simulink model "g729_enc_test_bench"  (R2013b)
settings: Solver=ode45  StartTime=0.0  StopTime=10000  RelTol=1e-3
PreLoadFcn:
  | g729_init
values from neighbouring files (symbols this model uses):
  fpga_up_rate = 20    [g729_init.m]
libraries: xbsIndex_r4 x50
settings Model: Creator=asubbiah  LastModifiedBy=asubbiah

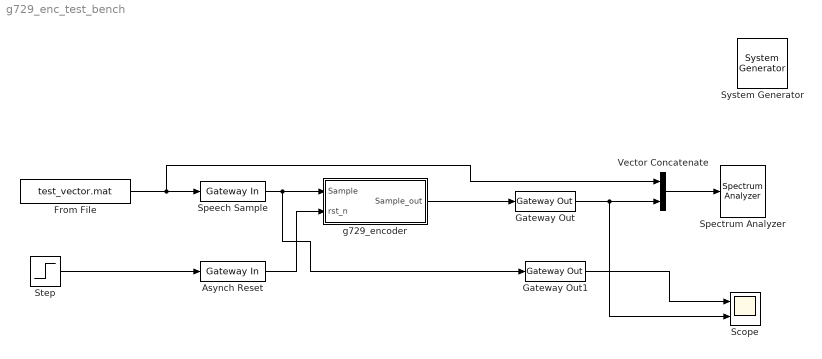
== system g729_enc_test_bench ==
  " System Generator" : xbsIndex_r4/ System Generator  Tag=genX  xilinxfamily=kintex7  part=xc7k325t  speed=-3  package=fbg676  synthesis_tool=Vivado  clock_wrapper=Clock Enables  directory=./netlist  proj_type=Vivado  Synth_file=Vivado Synthesis Defaults  Impl_file=Vivado Implementation Defaults  testbench=off  simulink_period=1/fpga_up_rate*2  sysclk_period=100  dcm_input_clock_period=10  incr_netlist=off  trim_vbits=Everywhere in SubSystem  dbl_ovrd=According to Block Masks  core_generation=According to Block Masks  run_coregen=off  deprecated_control=off  eval_field=0  block_type=sysgen
  Asynch Reset : xbsIndex_r4/Gateway In  gui_display_data_type=Boolean  arith_type=Boolean  n_bits=fixed_point  bin_pt=fixed_point_frac  preci_type=Single  exp_width=8  frac_width=24  quantization="Round  (unbiased: +/- Inf)"  overflow=Saturate  period=1  UseAsADC=off  ADCChannel='1'  interface=None  automatic_assignment=on  address_offset=hex2dec('00')  intf_description=''  timing_constraint=None  locs_specified=off  LOCs={}  io_standard={}  inherit_from_input=off  hdl_port=on  dbl_ovrd=off  block_type=gatewayin
  From File : FromFile  FileName=test_vector.mat  SampleTime=64
  Gateway Out : xbsIndex_r4/Gateway Out  inherit_from_input=off  hdl_port=on  rows=1  columns=1  UseAsDAC=off  DACChannel='1'  interface=None  automatic_assignment=on  address_offset=hex2dec('00')  intf_description=''  timing_constraint=None  locs_specified=off  LOCs={}  io_standard={}  block_type=gatewayout
  Gateway Out1 : xbsIndex_r4/Gateway Out  inherit_from_input=off  hdl_port=on  rows=1  columns=1  UseAsDAC=off  DACChannel='1'  interface=None  automatic_assignment=on  address_offset=hex2dec('00')  intf_description=''  timing_constraint=None  locs_specified=off  LOCs={}  io_standard={}  block_type=gatewayout
  Scope : Scope  NumInputPorts=2
      settings: YMin=-0.75~-1.2  YMax=0.75~0.2  MaxDataPoints=50000
  Spectrum Analyzer : SpectrumAnalyzer
      settings: CopyFcn=scopeextensions.ScopeBlock.onCoreBlockCopy(gcbh);  DeleteFcn=scopeextensions.ScopeBlock.callback(gcbh, 'onBlockDelete');  PreSaveFcn=scopeextensions.ScopeBlock.callback(gcbh, 'onModelSave');  NameChangeFcn=scopeextensions.ScopeBlock.callback(gcbh, 'onBlockRename');  DestroyFcn=scopeextensions.ScopeBlock.onBlockDestroy(gcbh)  CloseFcn=scopeextensions.ScopeBlock.callback(gcbh, 'onBlockClose');  PreDeleteFcn=scopeextensions.ScopeBlock.callback(gcbh, 'onBlockPreDelete');
  Speech Sample : xbsIndex_r4/Gateway In  gui_display_data_type=Fixed-point  arith_type="Signed  (2's comp)"  n_bits=fixed_point  bin_pt=fixed_point_frac  preci_type=Single  exp_width=8  frac_width=24  quantization="Round  (unbiased: +/- Inf)"  overflow=Saturate  period=1  UseAsADC=off  ADCChannel='1'  interface=None  automatic_assignment=on  address_offset=hex2dec('00')  intf_description=''  timing_constraint=None  locs_specified=off  LOCs={}  io_standard={}  inherit_from_input=off  hdl_port=on  dbl_ovrd=off  block_type=gatewayin
  Step : Step  SampleTime=0
  Vector Concatenate : Concatenate  Mode=Multidimensional array  ConcatenateDimension=2
  g729_encoder : Subsystem
  wires:
  Step/1 -> Asynch Reset/1
  From File/1 -> Vector Concatenate/1, Speech Sample/1
  Speech Sample/1 -> Gateway Out1/1, g729_encoder/1(Sample)
  Asynch Reset/1 -> g729_encoder/2(rst_n)
  g729_encoder/1(Sample_out) -> Gateway Out/1
  Gateway Out/1 -> Scope/2, Vector Concatenate/2
  Vector Concatenate/1 -> Spectrum Analyzer/1
  Gateway Out1/1 -> Scope/1

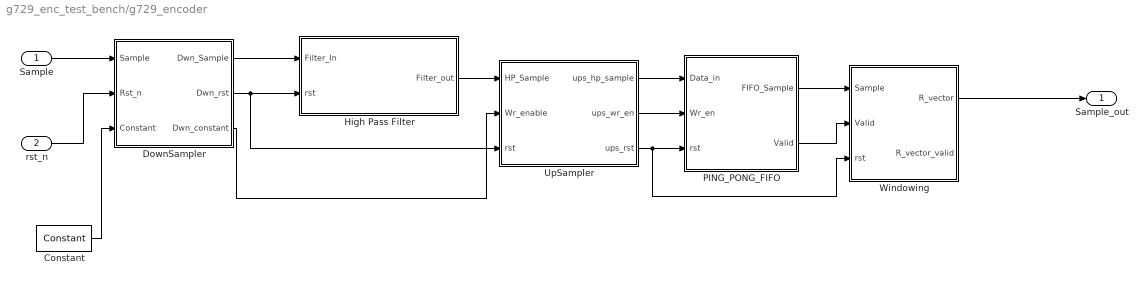
== system g729_enc_test_bench/g729_encoder ==
  Sample : Inport
  rst_n : Inport  Port=2
  Constant : xbsIndex_r4/Constant  const=1  gui_display_data_type=Boolean  arith_type=Boolean  n_bits=16  bin_pt=14  preci_type=Single  exp_width=8  frac_width=24  explicit_period=on  period=1  equ=P=C  opselect=C  inp2=PCIN>>17  opr=+  inp1=P  carry=CIN  dbl_ovrd=off  block_type=constant
  DownSampler : Subsystem
  High Pass Filter : Subsystem
  PING_PONG_FIFO : Subsystem
  UpSampler : Subsystem
  Windowing : Subsystem
  Sample_out : Outport
  wires:
  Sample/1 -> DownSampler/1(Sample)
  DownSampler/1(Dwn_Sample) -> High Pass Filter/1(Filter_In)
  DownSampler/2(Dwn_rst) -> High Pass Filter/2(rst), UpSampler/3(rst)
  rst_n/1 -> DownSampler/2(Rst_n)
  Constant/1 -> DownSampler/3(Constant)
  High Pass Filter/1(Filter_out) -> UpSampler/1(HP_Sample)
  UpSampler/1(ups_hp_sample) -> PING_PONG_FIFO/1(Data_in)
  UpSampler/2(ups_wr_en) -> PING_PONG_FIFO/2(Wr_en)
  DownSampler/3(Dwn_constant) -> UpSampler/2(Wr_enable)
  UpSampler/3(ups_rst) -> PING_PONG_FIFO/3(rst), Windowing/3(rst)
  PING_PONG_FIFO/1(FIFO_Sample) -> Windowing/1(Sample)
  PING_PONG_FIFO/2(Valid) -> Windowing/2(Valid)
  Windowing/1(R_vector) -> Sample_out/1

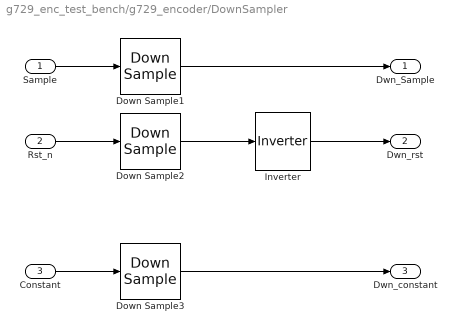
== system g729_enc_test_bench/g729_encoder/DownSampler ==
  Sample : Inport
  Rst_n : Inport  Port=2
  Constant : Inport  Port=3
  Down Sample1 : xbsIndex_r4/Down Sample  sample_ratio=2  sample_phase="Last Value of Frame  (most efficient)"  en=off  rst=off  latency=2  dbl_ovrd=off  block_type=dsamp
  Down Sample2 : xbsIndex_r4/Down Sample  sample_ratio=2  sample_phase="Last Value of Frame  (most efficient)"  en=off  rst=off  latency=2  dbl_ovrd=off  block_type=dsamp
  Down Sample3 : xbsIndex_r4/Down Sample  sample_ratio=2  sample_phase="Last Value of Frame  (most efficient)"  en=off  rst=off  latency=2  dbl_ovrd=off  block_type=dsamp
  Inverter : xbsIndex_r4/Inverter  en=off  latency=0  dbl_ovrd=off  block_type=inv
  Dwn_Sample : Outport
  Dwn_rst : Outport  Port=2
  Dwn_constant : Outport  Port=3
  wires:
  Sample/1 -> Down Sample1/1
  Down Sample1/1 -> Dwn_Sample/1
  Rst_n/1 -> Down Sample2/1
  Down Sample2/1 -> Inverter/1
  Inverter/1 -> Dwn_rst/1
  Constant/1 -> Down Sample3/1
  Down Sample3/1 -> Dwn_constant/1

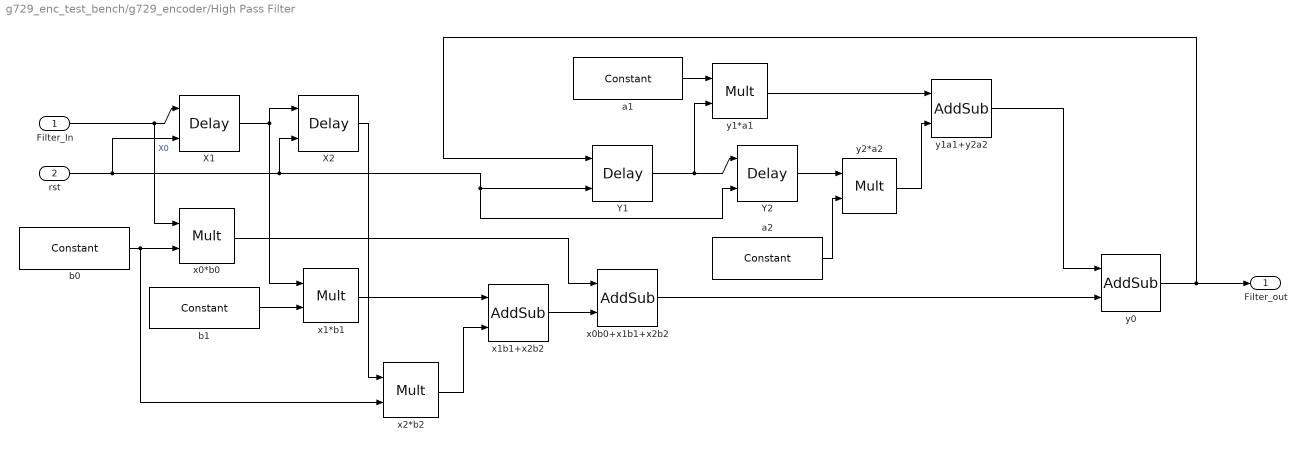
== system g729_enc_test_bench/g729_encoder/High Pass Filter ==
  Filter_In : Inport
  rst : Inport  Port=2
  X1 : xbsIndex_r4/Delay  rst=on  infoeditControl=Selection of Reset will increase slice count due to use of real FFs and instead of SRLs  en=off  latency=1  reg_retiming=off  dbl_ovrd=off  block_type=delay
  X2 : xbsIndex_r4/Delay  rst=on  infoeditControl=Selection of Reset will increase slice count due to use of real FFs and instead of SRLs  en=off  latency=1  reg_retiming=off  dbl_ovrd=off  block_type=delay
  Y1 : xbsIndex_r4/Delay  rst=on  infoeditControl=Selection of Reset will increase slice count due to use of real FFs and instead of SRLs  en=off  latency=1  reg_retiming=off  dbl_ovrd=off  block_type=delay
  Y2 : xbsIndex_r4/Delay  rst=on  infoeditControl=Selection of Reset will increase slice count due to use of real FFs and instead of SRLs  en=off  latency=1  reg_retiming=off  dbl_ovrd=off  block_type=delay
  a1 : xbsIndex_r4/Constant  const=1.9059465  gui_display_data_type=Fixed-point  arith_type=Signed (2's comp)  n_bits=fixed_point  bin_pt=fixed_point_frac  preci_type=Single  exp_width=8  frac_width=24  explicit_period=off  period=1  equ=P=C  opselect=C  inp2=PCIN>>17  opr=+  inp1=P  carry=CIN  dbl_ovrd=off  block_type=constant
  a2 : xbsIndex_r4/Constant  const=-0.91140240  gui_display_data_type=Fixed-point  arith_type=Signed (2's comp)  n_bits=fixed_point  bin_pt=fixed_point_frac  preci_type=Single  exp_width=8  frac_width=24  explicit_period=off  period=1  equ=P=C  opselect=C  inp2=PCIN>>17  opr=+  inp1=P  carry=CIN  dbl_ovrd=off  block_type=constant
  b0 : xbsIndex_r4/Constant  const=0.46363718  gui_display_data_type=Fixed-point  arith_type=Signed (2's comp)  n_bits=fixed_point  bin_pt=fixed_point_frac  preci_type=Single  exp_width=8  frac_width=24  explicit_period=off  period=1  equ=P=C  opselect=C  inp2=PCIN>>17  opr=+  inp1=P  carry=CIN  dbl_ovrd=off  block_type=constant
  b1 : xbsIndex_r4/Constant  const=-0.92724705  gui_display_data_type=Fixed-point  arith_type=Signed (2's comp)  n_bits=fixed_point  bin_pt=fixed_point_frac  preci_type=Single  exp_width=8  frac_width=24  explicit_period=off  period=1  equ=P=C  opselect=C  inp2=PCIN>>17  opr=+  inp1=P  carry=CIN  dbl_ovrd=off  block_type=constant
  x0*b0 : xbsIndex_r4/Mult  precision=User Defined  arith_type="Signed  (2's comp)"  n_bits=fixed_point  bin_pt=fixed_point_frac  quantization=Truncate  overflow=Wrap  en=off  latency=0  use_behavioral_HDL=off  opt=Speed  use_embedded=on  optimum_pipeline=off  pipeline=on  dbl_ovrd=off  use_rpm=on  placement_style=Triangular  block_type=mult
  x0b0+x1b1+x2b2 : xbsIndex_r4/AddSub  mode=Addition  use_carryin=off  use_carryout=off  en=off  latency=0  precision=Full  arith_type=Unsigned  n_bits=16  bin_pt=14  quantization=Truncate  overflow=Wrap  use_behavioral_HDL=off  hw_selection=Fabric  pipelined=on  dbl_ovrd=off  block_type=addsub
  x1*b1 : xbsIndex_r4/Mult  precision=User Defined  arith_type="Signed  (2's comp)"  n_bits=fixed_point  bin_pt=fixed_point_frac  quantization=Truncate  overflow=Wrap  en=off  latency=0  use_behavioral_HDL=off  opt=Speed  use_embedded=on  optimum_pipeline=off  pipeline=on  dbl_ovrd=off  use_rpm=on  placement_style=Triangular  block_type=mult
  x1b1+x2b2 : xbsIndex_r4/AddSub  mode=Addition  use_carryin=off  use_carryout=off  en=off  latency=0  precision=Full  arith_type=Unsigned  n_bits=16  bin_pt=14  quantization=Truncate  overflow=Wrap  use_behavioral_HDL=off  hw_selection=Fabric  pipelined=on  dbl_ovrd=off  block_type=addsub
  x2*b2 : xbsIndex_r4/Mult  precision=User Defined  arith_type="Signed  (2's comp)"  n_bits=fixed_point  bin_pt=fixed_point_frac  quantization=Truncate  overflow=Wrap  en=off  latency=0  use_behavioral_HDL=off  opt=Speed  use_embedded=on  optimum_pipeline=off  pipeline=on  dbl_ovrd=off  use_rpm=on  placement_style=Triangular  block_type=mult
  y0 : xbsIndex_r4/AddSub  mode=Addition  use_carryin=off  use_carryout=off  en=off  latency=0  precision=Full  arith_type=Unsigned  n_bits=16  bin_pt=14  quantization=Truncate  overflow=Wrap  use_behavioral_HDL=off  hw_selection=Fabric  pipelined=on  dbl_ovrd=off  block_type=addsub
  y1*a1 : xbsIndex_r4/Mult  precision=User Defined  arith_type="Signed  (2's comp)"  n_bits=fixed_point  bin_pt=fixed_point_frac  quantization=Truncate  overflow=Wrap  en=off  latency=0  use_behavioral_HDL=off  opt=Speed  use_embedded=on  optimum_pipeline=off  pipeline=on  dbl_ovrd=off  use_rpm=on  placement_style=Triangular  block_type=mult
  y1a1+y2a2 : xbsIndex_r4/AddSub  mode=Addition  use_carryin=off  use_carryout=off  en=off  latency=0  precision=Full  arith_type=Unsigned  n_bits=16  bin_pt=14  quantization=Truncate  overflow=Wrap  use_behavioral_HDL=off  hw_selection=Fabric  pipelined=on  dbl_ovrd=off  block_type=addsub
  y2*a2 : xbsIndex_r4/Mult  precision=User Defined  arith_type="Signed  (2's comp)"  n_bits=fixed_point  bin_pt=fixed_point_frac  quantization=Truncate  overflow=Wrap  en=off  latency=0  use_behavioral_HDL=off  opt=Speed  use_embedded=on  optimum_pipeline=off  pipeline=on  dbl_ovrd=off  use_rpm=on  placement_style=Triangular  block_type=mult
  Filter_out : Outport
  wires:
  rst/1 -> X1/2, X2/2, Y2/2, Y1/2
  y0/1 -> Filter_out/1, Y1/1
  y1a1+y2a2/1 -> y0/1
  x0b0+x1b1+x2b2/1 -> y0/2
  Y2/1 -> y2*a2/1
  a2/1 -> y2*a2/2
  y2*a2/1 -> y1a1+y2a2/2
  y1*a1/1 -> y1a1+y2a2/1
  a1/1 -> y1*a1/1
  Y1/1 -> y1*a1/2, Y2/1
  x2*b2/1 -> x1b1+x2b2/2
  x1*b1/1 -> x1b1+x2b2/1
  x0*b0/1 -> x0b0+x1b1+x2b2/1
  x1b1+x2b2/1 -> x0b0+x1b1+x2b2/2
  b0/1 -> x0*b0/2, x2*b2/2
  X2/1 -> x2*b2/1
  b1/1 -> x1*b1/2
  X1/1 -> x1*b1/1, X2/1
  Filter_In/1 -> X1/1, x0*b0/1  "X0"

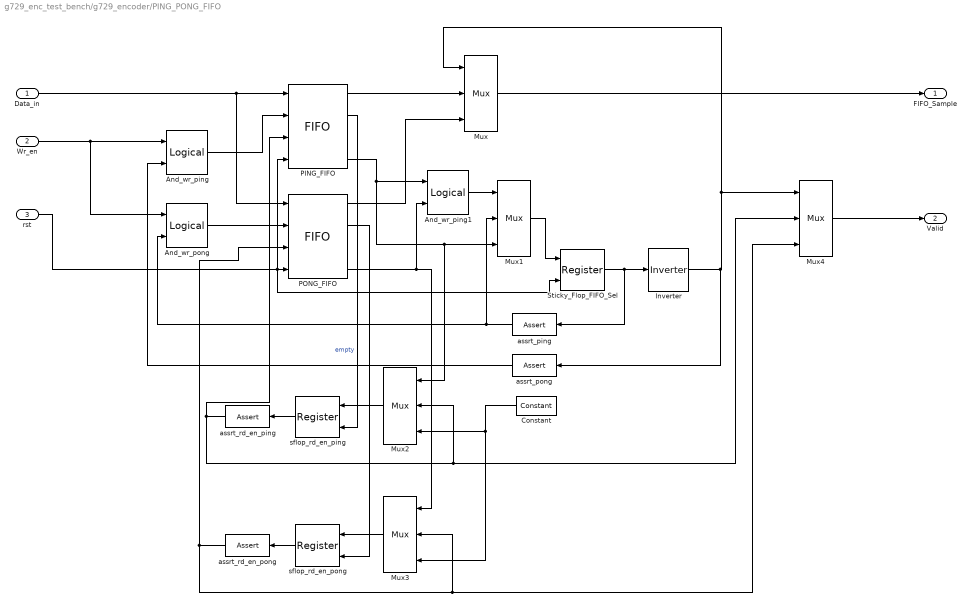
== system g729_enc_test_bench/g729_encoder/PING_PONG_FIFO ==
  Data_in : Inport
  Wr_en : Inport  Port=2
  rst : Inport  Port=3
  And_wr_ping : xbsIndex_r4/Logical  logical_function=AND  inputs=2  en=off  latency=0  precision=Full  arith_type=Unsigned  n_bits=16  bin_pt=0  align_bp=on  dbl_ovrd=off  block_type=logical
  And_wr_ping1 : xbsIndex_r4/Logical  logical_function=OR  inputs=2  en=off  latency=0  precision=Full  arith_type=Unsigned  n_bits=16  bin_pt=0  align_bp=on  dbl_ovrd=off  block_type=logical
  And_wr_pong : xbsIndex_r4/Logical  logical_function=AND  inputs=2  en=off  latency=0  precision=Full  arith_type=Unsigned  n_bits=16  bin_pt=0  align_bp=on  dbl_ovrd=off  block_type=logical
  Constant : xbsIndex_r4/Constant  const=1  gui_display_data_type=Boolean  arith_type=Boolean  n_bits=16  bin_pt=14  preci_type=Single  exp_width=8  frac_width=24  explicit_period=off  period=1  equ=P=C  opselect=C  inp2=PCIN>>17  opr=+  inp1=P  carry=CIN  dbl_ovrd=off  block_type=constant
  Inverter : xbsIndex_r4/Inverter  en=off  latency=0  dbl_ovrd=off  block_type=inv
  Mux{,1..4} (5 alike) : xbsIndex_r4/Mux  inputs=2  en=off  latency=0  precision=Full  arith_type=Unsigned  n_bits=16  bin_pt=14  quantization=Truncate  overflow=Wrap  dbl_ovrd=off  block_type=mux
  PING_FIFO : xbsIndex_r4/FIFO  mem_type=Block RAM  performance_options=Standard_FIFO  embedded_registers=off  depth=256  percent_nbits=1  rst=on  rst_latency=1  en=off  use_dcount=off  use_percent_full_port=off  use_almost_empty=off  almost_empty_thresh=2  use_almost_full=on  almost_full_thresh=fifo_stage1_thres  explicit_period=off  dbl_ovrd=off  block_type=fifo
  PONG_FIFO : xbsIndex_r4/FIFO  mem_type=Block RAM  performance_options=Standard_FIFO  embedded_registers=off  depth=256  percent_nbits=1  rst=on  rst_latency=1  en=off  use_dcount=off  use_percent_full_port=off  use_almost_empty=off  almost_empty_thresh=2  use_almost_full=on  almost_full_thresh=fifo_stage1_thres  explicit_period=off  dbl_ovrd=off  block_type=fifo
  Sticky_Flop_FIFO_Sel : xbsIndex_r4/Register  init=0  rst=on  en=off  dbl_ovrd=off  block_type=register
  assrt_ping : xbsIndex_r4/Assert  assert_type=off  type_source=Explicitly  gui_display_data_type=Boolean  arith_type=Boolean  n_bits=16  bin_pt=14  preci_type=Single  exp_width=8  frac_width=24  assert_rate=off  rate_source=Explicitly  period=1  output_port=on  block_type=assert
  assrt_pong : xbsIndex_r4/Assert  assert_type=off  type_source=Explicitly  gui_display_data_type=Boolean  arith_type=Boolean  n_bits=16  bin_pt=14  preci_type=Single  exp_width=8  frac_width=24  assert_rate=off  rate_source=Explicitly  period=1  output_port=on  block_type=assert
  assrt_rd_en_ping : xbsIndex_r4/Assert  assert_type=off  type_source=Explicitly  gui_display_data_type=Boolean  arith_type=Boolean  n_bits=16  bin_pt=14  preci_type=Single  exp_width=8  frac_width=24  assert_rate=off  rate_source=Explicitly  period=1  output_port=on  block_type=assert
  assrt_rd_en_pong : xbsIndex_r4/Assert  assert_type=off  type_source=Explicitly  gui_display_data_type=Boolean  arith_type=Boolean  n_bits=16  bin_pt=14  preci_type=Single  exp_width=8  frac_width=24  assert_rate=off  rate_source=Explicitly  period=1  output_port=on  block_type=assert
  sflop_rd_en_ping : xbsIndex_r4/Register  init=0  rst=on  en=off  dbl_ovrd=off  block_type=register
  sflop_rd_en_pong : xbsIndex_r4/Register  init=0  rst=on  en=off  dbl_ovrd=off  block_type=register
  FIFO_Sample : Outport
  Valid : Outport  Port=2
  wires:
  rst/1 -> Sticky_Flop_FIFO_Sel/2, PING_FIFO/4, PONG_FIFO/4
  Data_in/1 -> PONG_FIFO/1, PING_FIFO/1
  Wr_en/1 -> And_wr_pong/1, And_wr_ping/1
  Sticky_Flop_FIFO_Sel/1 -> assrt_ping/1, Inverter/1
  Inverter/1 -> assrt_pong/1, Mux4/1, Mux/1
  And_wr_ping/1 -> PING_FIFO/2
  PING_FIFO/1 -> Mux/2
  PONG_FIFO/1 -> Mux/3
  Mux/1 -> FIFO_Sample/1
  And_wr_pong/1 -> PONG_FIFO/2
  Mux1/1 -> Sticky_Flop_FIFO_Sel/1
  PING_FIFO/4 -> And_wr_ping1/1, Mux2/1, Mux1/3
  And_wr_ping1/1 -> Mux1/1
  PONG_FIFO/4 -> Mux3/1, And_wr_ping1/2
  Mux2/1 -> sflop_rd_en_ping/1
  PING_FIFO/2 -> sflop_rd_en_ping/2  "empty"
  sflop_rd_en_ping/1 -> assrt_rd_en_ping/1
  assrt_rd_en_ping/1 -> Mux2/2, Mux4/2, PING_FIFO/3
  assrt_ping/1 -> And_wr_pong/2, Mux1/2
  assrt_pong/1 -> And_wr_ping/2
  Mux3/1 -> sflop_rd_en_pong/1
  sflop_rd_en_pong/1 -> assrt_rd_en_pong/1
  assrt_rd_en_pong/1 -> Mux3/2, Mux4/3, PONG_FIFO/3
  Mux4/1 -> Valid/1
  PONG_FIFO/2 -> sflop_rd_en_pong/2
  Constant/1 -> Mux2/3, Mux3/3

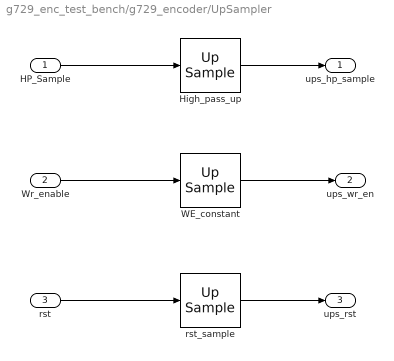
== system g729_enc_test_bench/g729_encoder/UpSampler ==
  HP_Sample : Inport
  Wr_enable : Inport  Port=2
  rst : Inport  Port=3
  High_pass_up : xbsIndex_r4/Up Sample  sample_ratio=fpga_up_rate  copy_samples=on  en=off  latency=1  dbl_ovrd=off  block_type=usamp
  WE_constant : xbsIndex_r4/Up Sample  sample_ratio=fpga_up_rate  copy_samples=off  en=off  latency=1  dbl_ovrd=off  block_type=usamp
  rst_sample : xbsIndex_r4/Up Sample  sample_ratio=fpga_up_rate  copy_samples=off  en=off  latency=1  dbl_ovrd=off  block_type=usamp
  ups_hp_sample : Outport
  ups_wr_en : Outport  Port=2
  ups_rst : Outport  Port=3
  wires:
  HP_Sample/1 -> High_pass_up/1
  High_pass_up/1 -> ups_hp_sample/1
  rst_sample/1 -> ups_rst/1
  rst/1 -> rst_sample/1
  WE_constant/1 -> ups_wr_en/1
  Wr_enable/1 -> WE_constant/1

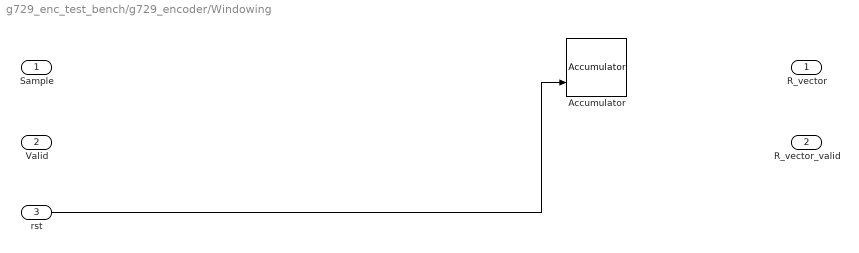
== system g729_enc_test_bench/g729_encoder/Windowing ==
  Sample : Inport
  Valid : Inport  Port=2
  rst : Inport  Port=3
  Accumulator : xbsIndex_r4/Accumulator  operation=Add  n_bits=8  overflow=Wrap  scale=1  rst=on  hasbypass=off  infoeditControl=reset for floating point data type must be asserted for a minimum of 2 cycles  en=off  latency=1  msb_inp=100  msb=100  lsb=-100  use_behavioral_HDL=on  implementation=Fabric  dbl_ovrd=off  block_type=accum
  R_vector : Outport
  R_vector_valid : Outport  Port=2
  wires:
  rst/1 -> Accumulator/2
